simulink model "MPC_CONTROLLER"  (R2022b)
settings: Solver=FixedStepAuto  StartTime=0.0  StopTime=250  FixedStep=0.1  RelTol=1e-3
values from neighbouring files (symbols this model uses):
  mpc_params_for_simulink = mpc_params    [MAIN_MPC.m]
  trajectory = generateTimedTrajectoryMPC(waypoints, velocities, distances,                                             time_vector, wheelbase, actual_duration)    [MAIN_MPC.m]
libraries: robotmobilelib x1
settings Model: Creator=emanuela  LastModifiedBy=emanuela
settings DataIOCC: ReturnWorkspaceOutputs=off

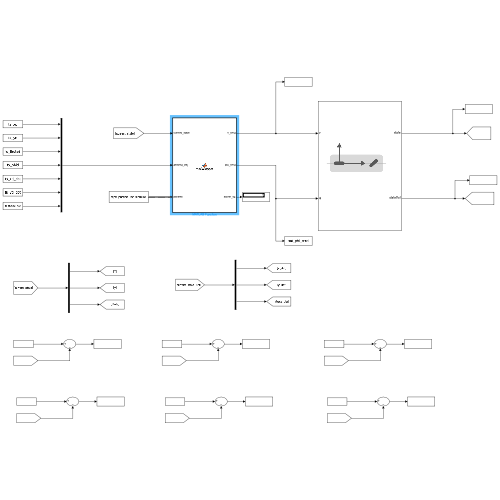
[thumbnail: Simulink's stored preview of the top-level diagram]
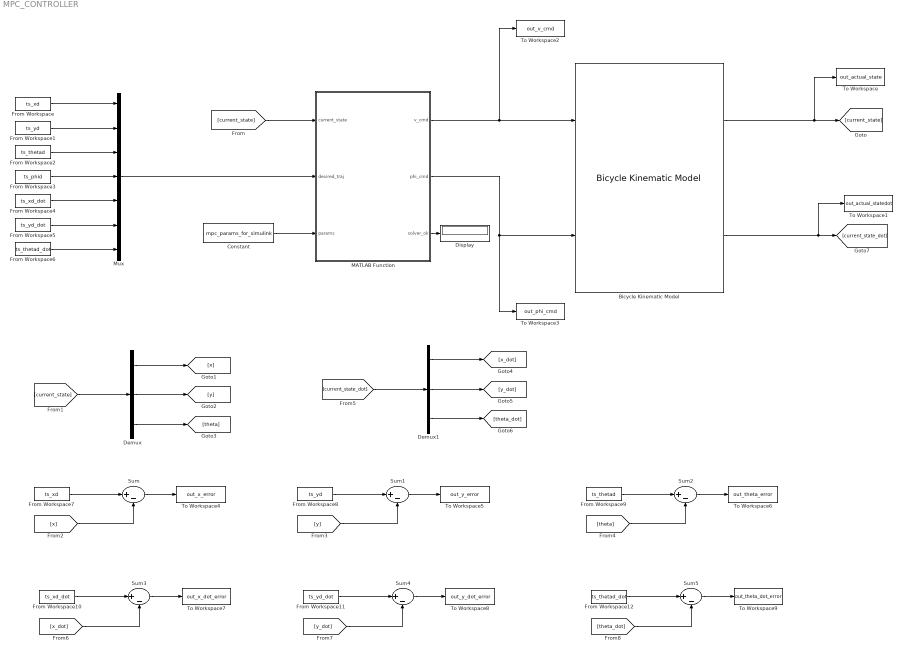
== system MPC_CONTROLLER ==
  Bicycle Kinematic Model : robotmobilelib/Bicycle Kinematic Model  VehicleInputs=Vehicle Speed & Steering Angle  WheelBase=L  VehicleSpeedRange=[0 2]  MaxSteeringAngle=pi/6  InitialState=[trajectory.xd(1), trajectory.yd(1), trajectory.thetad(1)]  SimulateUsing=Interpreted execution
  Constant : Constant  Value=mpc_params_for_simulink  OutDataTypeStr=Bus: mpc_params_bus
  Demux : Demux  Outputs=3
  Demux1 : Demux  Outputs=3
  Display : Display
  From Workspace : FromWorkspace  VariableName=ts_xd
  From Workspace1 : FromWorkspace  VariableName=ts_yd
  From Workspace10 : FromWorkspace  VariableName=ts_xd_dot
  From Workspace11 : FromWorkspace  VariableName=ts_yd_dot
  From Workspace12 : FromWorkspace  VariableName=ts_thetad_dot
  From Workspace2 : FromWorkspace  VariableName=ts_thetad
  From Workspace3 : FromWorkspace  VariableName=ts_phid
  From Workspace4 : FromWorkspace  VariableName=ts_xd_dot
  From Workspace5 : FromWorkspace  VariableName=ts_yd_dot
  From Workspace6 : FromWorkspace  VariableName=ts_thetad_dot
  From Workspace7 : FromWorkspace  VariableName=ts_xd
  From Workspace8 : FromWorkspace  VariableName=ts_yd
  From Workspace9 : FromWorkspace  VariableName=ts_thetad
  MATLAB Function : MATLAB Function  TreatAsAtomicUnit=on
  Mux : Mux  Inputs=7
  Sum{,1..5} (6 alike) : Sum  Inputs=|+-
  To Workspace : ToWorkspace  VariableName=out_actual_state  SaveFormat=Timeseries  SampleTime=-1
  To Workspace1 : ToWorkspace  VariableName=out_actual_statedot  SaveFormat=Timeseries  SampleTime=-1
  To Workspace2 : ToWorkspace  VariableName=out_v_cmd  SaveFormat=Timeseries  SampleTime=-1
  To Workspace3 : ToWorkspace  VariableName=out_phi_cmd  SaveFormat=Timeseries  SampleTime=-1
  To Workspace4 : ToWorkspace  VariableName=out_x_error  SaveFormat=Timeseries  SampleTime=-1
  To Workspace5 : ToWorkspace  VariableName=out_y_error  SaveFormat=Timeseries  SampleTime=-1
  To Workspace6 : ToWorkspace  VariableName=out_theta_error  SaveFormat=Timeseries  SampleTime=-1
  To Workspace7 : ToWorkspace  VariableName=out_x_dot_error  SaveFormat=Timeseries  SampleTime=-1
  To Workspace8 : ToWorkspace  VariableName=out_y_dot_error  SaveFormat=Timeseries  SampleTime=-1
  To Workspace9 : ToWorkspace  VariableName=out_theta_dot_error  SaveFormat=Timeseries  SampleTime=-1
  wires:
  From Workspace2/1 -> Mux/3
  From Workspace4/1 -> Mux/5
  From Workspace3/1 -> Mux/4
  MATLAB Function/2(phi_cmd) -> To Workspace3/1, Bicycle Kinematic Model/2
  From Workspace5/1 -> Mux/6
  Constant/1 -> MATLAB Function/3(params)
  MATLAB Function/1(v_cmd) -> To Workspace2/1, Bicycle Kinematic Model/1
  Bicycle Kinematic Model/1 -> [current_state], To Workspace/1
  From Workspace/1 -> Mux/1
  From Workspace6/1 -> Mux/7
  From Workspace1/1 -> Mux/2
  Mux/1 -> MATLAB Function/2(desired_traj)
  Demux/1 -> [x]
  [x] -> Sum/2
  From Workspace7/1 -> Sum/1
  [current_state_dot] -> Demux1/1
  [theta_dot] -> Sum5/2
  [y] -> Sum1/2
  From Workspace9/1 -> Sum2/1
  [y_dot] -> Sum4/2
  [current_state] -> Demux/1
  From Workspace11/1 -> Sum4/1
  Sum4/1 -> To Workspace8/1
  [x_dot] -> Sum3/2
  [theta] -> Sum2/2
  Sum/1 -> To Workspace4/1
  Demux1/2 -> [y_dot]
  From Workspace10/1 -> Sum3/1
  Sum3/1 -> To Workspace7/1
  Sum1/1 -> To Workspace5/1
  Demux/3 -> [theta]
  Demux1/3 -> [theta_dot]
  Demux/2 -> [y]
  Sum2/1 -> To Workspace6/1
  Sum5/1 -> To Workspace9/1
  Demux1/1 -> [x_dot]
  From Workspace8/1 -> Sum1/1
  From Workspace12/1 -> Sum5/1
  Bicycle Kinematic Model/2 -> To Workspace1/1, [current_state_dot]
  [current_state] -> MATLAB Function/1(current_state)
  MATLAB Function/3(solver_ok) -> Display/1

== matlab function MPC_CONTROLLER/MATLAB Function ==
  settings: updateMethod=DISCRETE  sampleTime=0.1
  data: current_state input; v_cmd output; desired_traj input; params input; phi_cmd output; solver_ok output
function [v_cmd, phi_cmd, solver_ok] = mpcWrapper(current_state, desired_traj, params)
% Simulink MATLAB Function Block Wrapper for MPC Controller
% 
% Modified version with solver_ok output for monitoring optimization status
%
% Inputs:
%   current_state: [3×1 double] - [x, y, theta] current vehicle state
%   desired_traj: [7×1 double] - [xd, yd, thetad, phid, xd_dot, yd_dot, thetad_dot]
%   params: struct - controller parameters from bus object
%
% Outputs:
%   v_cmd: [1×1 double] - velocity command [m/s]
%   phi_cmd: [1×1 double] - steering angle command [rad]
%   solver_ok: [1×1 double] - solver status (1.0 = success, 0.0 = failure)

% Initialize output variables with default values
v_cmd = 0.0;
phi_cmd = 0.0;
solver_ok = 0.0;

% Call the main MPC controller function with all three outputs
[v_cmd, phi_cmd, solver_ok] = mpcController_Simulink(current_state, desired_traj, params);

end

function [v_cmd, phi_cmd, solver_ok] = mpcController_Simulink(current_state, desired_trajectory, controller_params)

mpc_params = controller_params;

%% INPUT VALIDATION
% Basic input validation
if length(current_state) < 3
    % Handle error - return safe defaults
    v_cmd = 0.0;
    phi_cmd = 0.0;
    solver_ok = 0.0;
    return;
end

if length(desired_trajectory) < 7
    % Handle error - return safe defaults
    v_cmd = 0.0;
    phi_cmd = 0.0;
    solver_ok = 0.0;
    return;
end

%% EXTRACT DATA
% Current vehicle state
x = current_state(1);
y = current_state(2);
theta = wrapToPi(current_state(3));

% Desired trajectory at current time
xd = desired_trajectory(1);
yd = desired_trajectory(2);
thetad = wrapToPi(desired_trajectory(3));
phid = desired_trajectory(4);
xd_dot = desired_trajectory(5);
yd_dot = desired_trajectory(6);
thetad_dot = desired_trajectory(7);

% Extract parameters
L = mpc_params.wheelbase;
Np = mpc_params.prediction_horizon;
dt = mpc_params.sampling_time;
Q_diag = mpc_params.Q_weights;
R_diag = mpc_params.R_weights;
v_max = mpc_params.v_max;
v_min = mpc_params.v_min;
phi_max = mpc_params.phi_max;
smoothing_factor = mpc_params.smoothing_factor;

%% PERSISTENT VARIABLES FOR SMOOTH CONTROL
persistent v_cmd_prev phi_cmd_prev init_flag
if isempty(init_flag)
    v_cmd_prev = 0.0;  % Start from zero velocity
    phi_cmd_prev = 0.0;
    init_flag = true;
end

%% COMPUTE ERRORS AND CHECK PARKING STATUS
% Global coordinate errors
ex_global = x - xd;
ey_global = y - yd;
etheta_global = wrapToPi(theta - thetad);

% Position error magnitude
position_error = sqrt(ex_global^2 + ey_global^2);

% Reference velocity
v_ref = sqrt(xd_dot^2 + yd_dot^2);

% Check if parking is complete
parking_complete = (position_error < 0.3) && (v_ref < 0.01);
approaching_target = (position_error < 2.0) && (v_ref < 0.5);

%% PARKING MODE LOGIC
if parking_complete
    % Parking complete: full stop
    v_cmd = 0.0;
    
    % Small heading correction if needed
    if abs(etheta_global) > 0.1  % ~5.7 degrees
        phi_cmd = -mpc_params.fallback_kp_heading * 0.5 * etheta_global;
    else
        phi_cmd = 0.0;
    end
    
    % Update persistent variables
    v_cmd_prev = 0.0;
    if abs(etheta_global) < 0.05
        phi_cmd_prev = 0.0;
    end
    
    solver_ok = 1.0;  % Parking logic successful
    return;  % Exit early
end

%% COMPUTE REFERENCE VELOCITY CONSIDERING PARKING
% If reference stopped but not at target, use position-based velocity
if v_ref < 0.01 && position_error > 0.5
    v_ref = min(1.0, position_error);  % Proportional to distance
end

% Limit reference velocity
v_ref = max(v_min, min(v_max, v_ref));

%% TRANSFORM ERRORS TO LOCAL COORDINATES
cos_thetad = cos(thetad);
sin_thetad = sin(thetad);

% Transform to local trajectory coordinates
e_lateral = -ex_global * sin_thetad + ey_global * cos_thetad;
e_longitudinal = ex_global * cos_thetad + ey_global * sin_thetad;
e_heading = etheta_global;

% State error vector
e_current = [e_lateral; e_longitudinal; e_heading];

%% ADAPTIVE MPC WEIGHTS FOR PARKING
% Modify weights based on situation
Q_adaptive = Q_diag;
R_adaptive = R_diag;

if approaching_target
    % Increase position tracking importance when close to target
    Q_adaptive(1) = Q_adaptive(1) * 2.0;  % Lateral error more important
    Q_adaptive(3) = Q_adaptive(3) * 1.5;  % Heading error more important
    R_adaptive(2) = R_adaptive(2) * 2.0;  % Smoother steering
end

%% MODEL LINEARIZATION
% Use actual reference velocity for linearization
v_lin = max(0.5, v_ref);  % Avoid singularities at low speed

% Continuous-time system matrices
A_cont = [0,    0,    v_lin;
          0,    0,    0;
          0,    0,    0];

B_cont = [0,    0;
          1,    0;
          0,    v_lin/L];

% Discrete-time system matrices
Ad = eye(3) + A_cont * dt;
Bd = B_cont * dt;

%% BUILD MPC OPTIMIZATION PROBLEM
% Weight matrices with adaptive values
Q = diag(Q_adaptive);
R = diag(R_adaptive);

% Build prediction matrices
Phi = zeros(3*Np, 3);
Gamma = zeros(3*Np, 2*Np);

% Build prediction matrices iteratively
Ad_power = Ad;
for i = 1:Np
    Phi(3*(i-1)+1:3*i, :) = Ad_power;
    
    Ad_temp = eye(3);
    for j = 1:i
        Gamma(3*(i-1)+1:3*i, 2*(j-1)+1:2*j) = Ad_temp * Bd;
        Ad_temp = Ad_temp * Ad;
    end
    
    Ad_power = Ad_power * Ad;
end

% Extended weight matrices
Q_bar = kron(eye(Np), Q);
R_bar = kron(eye(Np), R);

% Quadratic program formulation
H = 2 * (Gamma' * Q_bar * Gamma + R_bar);
f = 2 * Gamma' * Q_bar * Phi * e_current;

%% DEFINE OPERATIONAL CONSTRAINTS
% Adaptive constraints based on situation
if approaching_target
    % Tighter constraints when parking
    v_max_local = min(v_max, 1.0);
    phi_max_local = phi_max * 0.8;
else
    v_max_local = v_max;
    phi_max_local = phi_max;
end

% Control constraints
delta_v_max = v_max_local - v_ref;
delta_v_min = v_min - v_ref;
delta_phi_max = phi_max_local - phid;
delta_phi_min = -phi_max_local - phid;

% Constraint matrices
A_ineq = [eye(2*Np); -eye(2*Np)];
b_ineq = [repmat([delta_v_max; delta_phi_max], Np, 1);
          repmat([-delta_v_min; -delta_phi_min], Np, 1)];

%% SOLVE OPTIMIZATION PROBLEM
[U_opt, solve_success] = solveQP_Simple(H, f, A_ineq, b_ineq, 2*Np);

if solve_success
    solver_ok = 1.0;
    
    % Extract optimal control inputs
    delta_v_opt = U_opt(1);
    delta_phi_opt = U_opt(2);
    
    % Compute final commands
    v_cmd = v_ref + delta_v_opt;
    phi_cmd = phid + delta_phi_opt;
else
    solver_ok = 0.0;
    
    % Enhanced fallback controller for parking
    [v_cmd, phi_cmd] = computeEnhancedFallbackControl(e_current, v_ref, phid, ...
                                                      position_error, approaching_target, mpc_params);
end

%% APPLY SAFETY CONSTRAINTS AND PARKING LOGIC
% Apply approach speed reduction
if approaching_target
    approach_factor = max(0.1, (position_error - 0.3) / 1.7);
    v_cmd = v_cmd * approach_factor;
end

% Saturation
v_cmd = max(v_min, min(v_max, v_cmd));
phi_cmd = max(-phi_max, min(phi_max, phi_cmd));

%% RATE LIMITING FOR SMOOTH CONTROL
max_accel = 1.5;      % m/s^2
max_phi_rate = 0.8;   % rad/s

% Velocity rate limit
v_rate = (v_cmd - v_cmd_prev) / dt;
if abs(v_rate) > max_accel
    v_cmd = v_cmd_prev + sign(v_rate) * max_accel * dt;
end

% Steering rate limit
phi_rate = (phi_cmd - phi_cmd_prev) / dt;
if abs(phi_rate) > max_phi_rate
    phi_cmd = phi_cmd_prev + sign(phi_rate) * max_phi_rate * dt;
end

%% COMMAND SMOOTHING
% Adaptive smoothing based on speed
if v_cmd < 0.5
    % Less smoothing at low speed for better control
    alpha_v = 0.7;
    alpha_phi = 0.8;
else
    alpha_v = smoothing_factor;
    alpha_phi = smoothing_factor;
end

v_cmd = alpha_v * v_cmd + (1 - alpha_v) * v_cmd_prev;
phi_cmd = alpha_phi * phi_cmd + (1 - alpha_phi) * phi_cmd_prev;

% Update previous values
v_cmd_prev = v_cmd;
phi_cmd_prev = phi_cmd;

%% FINAL SAFETY CHECK
% Ensure stop when reference velocity is zero and close to target
if v_ref < 0.01 && position_error < 0.5
    v_cmd = 0.0;
    v_cmd_prev = 0.0;
end

end

%% AUXILIARY FUNCTIONS

function [v_cmd, phi_cmd] = computeEnhancedFallbackControl(e_current, v_ref, phi_ref, ...
                                                           position_error, approaching_target, params)
    % Enhanced fallback controller for parking scenarios
    
    e_lateral = e_current(1);
    e_longitudinal = e_current(2);
    e_heading = e_current(3);
    
    % Adaptive gains based on situation
    if approaching_target
        kp_long = params.fallback_kp_longitudinal * 0.5;
        kp_lat = params.fallback_kp_lateral * 1.5;
        kp_head = params.fallback_kp_heading * 1.2;
    else
        kp_long = params.fallback_kp_longitudinal;
        kp_lat = params.fallback_kp_lateral;
        kp_head = params.fallback_kp_heading;
    end
    
    % Velocity control with position feedback
    if v_ref < 0.1 && position_error > 0.5
        % Use position-based control when reference is nearly zero
        v_cmd = min(1.0, position_error);
    else
        v_cmd = v_ref + kp_long * e_longitudinal;
    end
    
    % Steering control
    phi_cmd = phi_ref - kp_lat * e_lateral - kp_head * e_heading;
    
    % Apply constraints
    v_cmd = max(params.v_min, min(params.v_max, v_cmd));
    phi_cmd = max(-params.phi_max, min(params.phi_max, phi_cmd));
end

function angle_diff = wrapToPi(angle)
    % Wrap angle to [-pi, pi] range
    angle_diff = atan2(sin(angle), cos(angle));
end

function [x, success] = solveQP_Simple(H, f, A, b, n)
    % Simplified QP solver compatible with code generation
    
    % Initialize
    x = zeros(n, 1);
    success = false;
    
    % Parameters
    max_iter = 30;
    tolerance = 1e-4;
    alpha = 0.05;
    
    % Regularize H matrix for numerical stability
    H_reg = H + 1e-6 * eye(size(H));
    
    for iter = 1:max_iter
        % Compute gradient
        grad = H_reg * x + f;
        
        % Gradient descent step
        x_new = x - alpha * grad;
        
        % Simple box constraint projection
        x_new = projectSimpleConstraints(x_new, n);
        
        % Check convergence
        if norm(x_new - x) < tolerance
            success = true;
            break;
        end
        
        x = x_new;
    end
    
    % Mark as successful if we've made progress
    if ~success && iter >= max_iter
        success = true;  % Accept the best solution found
    end
end

function x_proj = projectSimpleConstraints(x, n)
    % Simple projection for typical MPC constraints
    
    x_proj = x;
    
    % Typical bounds for velocity and steering deviations
    v_delta_max = 1.0;    % Maximum velocity deviation
    phi_delta_max = 0.3;  % Maximum steering deviation
    
    % Project velocity deviations
    for i = 1:2:n
        x_proj(i) = max(-v_delta_max, min(v_delta_max, x_proj(i)));
    end
    
    % Project steering deviations
    for i = 2:2:n
        x_proj(i) = max(-phi_delta_max, min(phi_delta_max, x_proj(i)));
    end
end
